simulink model "SimpleStateflow"  (Simulink 7.4)
settings: Solver=ode45  StartTime=0.0  StopTime=10.0  RelTol=1e-3
settings Model: Creator=dread  LastModifiedBy=dread

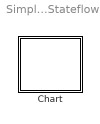
== system SimpleStateflow ==
  Chart : Stateflow chart

== stateflow chart Chart ==
  state Start
  state End
  Start -> End
  (default) -> Start
